simulink model "DataPath"  (R2025a)
settings: Solver=FixedStepAuto  StartTime=0  StopTime=0.02  FixedStep=1e-7  RelTol=1e-3
undefined symbols (not defined in the file): Bit_1, Bit_2, Bit_3, Bit_4, Bit_5, Bit_6, Bit_7, Bit_8
libraries: simulink_extras x126, fl_lib x34, nesl_utility x18, simulink x2
(part 6 of 7)

== system DataPath/Subsystem/ALU Regs/B2/Subsystem8 ==
  Data : Inport
  Store : Inport  Port=2
  Clock : Inport  Port=3
  Clear : Inport  Port=4
  AND : Logic  IconShape=distinctive  AllPortsSameDT=off  OutDataTypeStr=boolean
  AND1 : Logic  IconShape=distinctive  AllPortsSameDT=off  OutDataTypeStr=boolean
  D Flip-Flop : simulink_extras/Flip Flops/D Flip-Flop
  NOT : Logic  Operator=NOT  IconShape=distinctive  AllPortsSameDT=off  OutDataTypeStr=boolean
  NOT1 : Logic  Operator=NOT  IconShape=distinctive  AllPortsSameDT=off  OutDataTypeStr=boolean
  OR : Logic  Operator=OR  IconShape=distinctive  AllPortsSameDT=off  OutDataTypeStr=boolean
  Q : Outport
  !Q : Outport  Port=2
  wires:
  AND1/1 -> OR/2
  AND/1 -> OR/1
  D Flip-Flop/1 -> Q/1, AND1/2
  NOT/1 -> AND1/1
  Store/1 -> AND/2, NOT/1
  Clock/1 -> D Flip-Flop/2
  Data/1 -> AND/1
  OR/1 -> D Flip-Flop/1
  D Flip-Flop/2 -> !Q/1
  Clear/1 -> NOT1/1
  NOT1/1 -> D Flip-Flop/3

== system DataPath/Subsystem/Normalize Div/Subsystem1/Subsystem6 ==
  Data : Inport
  CLK : Inport  Port=2
  Delay One Step : Delay  DelayLength=1
  NAND{1..4} (4 alike) : Logic  Operator=NAND  IconShape=distinctive  AllPortsSameDT=off  OutDataTypeStr=boolean
  Q : Outport
  !Q : Outport  Port=2
  wires:
  NAND1/1 -> Delay One Step/1
  NAND4/1 -> NAND2/2
  Delay One Step/1 -> NAND2/1, Q/1  "Q"
  NAND2/1 -> !Q/1, NAND1/2
  NAND3/1 -> NAND4/1, NAND1/1
  CLK/1 -> NAND3/2, NAND4/2
  Data/1 -> NAND3/1

== system DataPath/Subsystem/Normalize Div/Subsystem1/Subsystem7 ==
  Data : Inport
  CLK : Inport  Port=2
  Delay One Step : Delay  DelayLength=1
  NAND{1..4} (4 alike) : Logic  Operator=NAND  IconShape=distinctive  AllPortsSameDT=off  OutDataTypeStr=boolean
  Q : Outport
  !Q : Outport  Port=2
  wires:
  NAND1/1 -> Delay One Step/1
  NAND4/1 -> NAND2/2
  Delay One Step/1 -> NAND2/1, Q/1  "Q"
  NAND2/1 -> !Q/1, NAND1/2
  NAND3/1 -> NAND4/1, NAND1/1
  CLK/1 -> NAND3/2, NAND4/2
  Data/1 -> NAND3/1

== system DataPath/Subsystem/Normalize Div/Subsystem8/Subsystem6 ==
  Data : Inport
  CLK : Inport  Port=2
  Delay One Step : Delay  DelayLength=1
  NAND{1..4} (4 alike) : Logic  Operator=NAND  IconShape=distinctive  AllPortsSameDT=off  OutDataTypeStr=boolean
  Q : Outport
  !Q : Outport  Port=2
  wires:
  NAND1/1 -> Delay One Step/1
  NAND4/1 -> NAND2/2
  Delay One Step/1 -> NAND2/1, Q/1  "Q"
  NAND2/1 -> !Q/1, NAND1/2
  NAND3/1 -> NAND4/1, NAND1/1
  CLK/1 -> NAND3/2, NAND4/2
  Data/1 -> NAND3/1

== system DataPath/Subsystem/Normalize Div/Subsystem8/Subsystem7 ==
  Data : Inport
  CLK : Inport  Port=2
  Delay One Step : Delay  DelayLength=1
  NAND{1..4} (4 alike) : Logic  Operator=NAND  IconShape=distinctive  AllPortsSameDT=off  OutDataTypeStr=boolean
  Q : Outport
  !Q : Outport  Port=2
  wires:
  NAND1/1 -> Delay One Step/1
  NAND4/1 -> NAND2/2
  Delay One Step/1 -> NAND2/1, Q/1  "Q"
  NAND2/1 -> !Q/1, NAND1/2
  NAND3/1 -> NAND4/1, NAND1/1
  CLK/1 -> NAND3/2, NAND4/2
  Data/1 -> NAND3/1

== system DataPath/Subsystem/Stepper/Subsystem1/DFF ==
  Data : Inport
  CLK : Inport  Port=2
  DLatch Master : Subsystem
  DLatch Slave : Subsystem
  NOT6 : Logic  Operator=NOT  IconShape=distinctive  AllPortsSameDT=off  OutDataTypeStr=boolean
  Q : Outport
  !Q : Outport  Port=2
  wires:
  DLatch Master/1(Q) -> DLatch Slave/1(Data)
  NOT6/1 -> DLatch Master/2(CLK)
  CLK/1 -> DLatch Slave/2(CLK), NOT6/1
  Data/1 -> DLatch Master/1(Data)
  DLatch Slave/1(Q) -> Q/1
  DLatch Slave/2(!Q) -> !Q/1

== system DataPath/Subsystem/Stepper/Subsystem2/DFF ==
  Data : Inport
  CLK : Inport  Port=2
  DLatch Master : Subsystem
  DLatch Slave : Subsystem
  NOT6 : Logic  Operator=NOT  IconShape=distinctive  AllPortsSameDT=off  OutDataTypeStr=boolean
  Q : Outport
  !Q : Outport  Port=2
  wires:
  DLatch Master/1(Q) -> DLatch Slave/1(Data)
  NOT6/1 -> DLatch Master/2(CLK)
  CLK/1 -> DLatch Slave/2(CLK), NOT6/1
  Data/1 -> DLatch Master/1(Data)
  DLatch Slave/1(Q) -> Q/1
  DLatch Slave/2(!Q) -> !Q/1

== system DataPath/Subsystem/Stepper/Subsystem3/DFF ==
  Data : Inport
  CLK : Inport  Port=2
  DLatch Master : Subsystem
  DLatch Slave : Subsystem
  NOT6 : Logic  Operator=NOT  IconShape=distinctive  AllPortsSameDT=off  OutDataTypeStr=boolean
  Q : Outport
  !Q : Outport  Port=2
  wires:
  DLatch Master/1(Q) -> DLatch Slave/1(Data)
  NOT6/1 -> DLatch Master/2(CLK)
  CLK/1 -> DLatch Slave/2(CLK), NOT6/1
  Data/1 -> DLatch Master/1(Data)
  DLatch Slave/1(Q) -> Q/1
  DLatch Slave/2(!Q) -> !Q/1

== system DataPath/Subsystem/Stepper/Subsystem4/DFF ==
  Data : Inport
  CLK : Inport  Port=2
  DLatch Master : Subsystem
  DLatch Slave : Subsystem
  NOT6 : Logic  Operator=NOT  IconShape=distinctive  AllPortsSameDT=off  OutDataTypeStr=boolean
  Q : Outport
  !Q : Outport  Port=2
  wires:
  DLatch Master/1(Q) -> DLatch Slave/1(Data)
  NOT6/1 -> DLatch Master/2(CLK)
  CLK/1 -> DLatch Slave/2(CLK), NOT6/1
  Data/1 -> DLatch Master/1(Data)
  DLatch Slave/1(Q) -> Q/1
  DLatch Slave/2(!Q) -> !Q/1

== system DataPath/Subsystem1/ALU/Adder & Logic Module/Subsystem1 ==
  Neg_A : Inport
  Carry In : Inport  Port=2
  B : Inport  Port=3
  A : Inport  Port=4
  Subtract : Inport  Port=5
  = So far : Inport  Port=6
  A>B Prev : Inport  Port=7
  !A : Logic  Operator=NOT  IconShape=distinctive  AllPortsSameDT=off  OutDataTypeStr=boolean
  !A^B : Logic  Operator=NOT  IconShape=distinctive  AllPortsSameDT=off  OutDataTypeStr=boolean
  !B : Logic  Operator=NOT  IconShape=distinctive  AllPortsSameDT=off  OutDataTypeStr=boolean
  3AND : Logic  Inputs=3  IconShape=distinctive  AllPortsSameDT=off  OutDataTypeStr=boolean
  A&&B : Logic  IconShape=distinctive  AllPortsSameDT=off  OutDataTypeStr=boolean
  A-Modifier : Logic  Operator=XOR  IconShape=distinctive  AllPortsSameDT=off  OutDataTypeStr=boolean
  ALN : Logic  Operator=OR  IconShape=distinctive  AllPortsSameDT=off  OutDataTypeStr=boolean
  A^B : Logic  Operator=XOR  IconShape=distinctive  AllPortsSameDT=off  OutDataTypeStr=boolean
  A||B : Logic  Operator=OR  IconShape=distinctive  AllPortsSameDT=off  OutDataTypeStr=boolean
  B-Modifier : Logic  Operator=XOR  IconShape=distinctive  AllPortsSameDT=off  OutDataTypeStr=boolean
  CE : Logic  IconShape=distinctive  AllPortsSameDT=off  OutDataTypeStr=boolean
  CI&&A^B : Logic  IconShape=distinctive  AllPortsSameDT=off  OutDataTypeStr=boolean
  CO|| : Logic  Operator=OR  IconShape=distinctive  AllPortsSameDT=off  OutDataTypeStr=boolean
  Mux : Mux  Inputs=6
  SUM : Logic  Operator=XOR  IconShape=distinctive  AllPortsSameDT=off  OutDataTypeStr=boolean
  Carry Out : Outport
  Bus : Outport  Port=2
  = Currently : Outport  Port=3
  A >B Next : Outport  Port=4
  wires:
  B/1 -> B-Modifier/1
  Subtract/1 -> B-Modifier/2
  CI&&A^B/1 -> CO||/1
  A&&B/1 -> Mux/2, CO||/2  "AND"
  CO||/1 -> Carry Out/1
  B-Modifier/1 -> A&&B/2, !B/1, A||B/2, A^B/2  "B_M"
  Carry In/1 -> CI&&A^B/2, SUM/2
  SUM/1 -> Mux/1  "Sum"
  A^B/1 -> Mux/4, CI&&A^B/1, 3AND/3, !A^B/1, SUM/1  "XOR"
  A>B Prev/1 -> ALN/1
  ALN/1 -> A >B Next/1
  !A^B/1 -> CE/2
  CE/1 -> = Currently/1
  3AND/1 -> ALN/2
  A-Modifier/1 -> 3AND/2, !A/1, A||B/1, A&&B/1, A^B/1
  = So far/1 -> CE/1, 3AND/1
  A||B/1 -> Mux/3  "OR"
  Mux/1 -> Bus/1
  !A/1 -> Mux/5  "!A"
  !B/1 -> Mux/6  "!B"
  A/1 -> A-Modifier/2
  Neg_A/1 -> A-Modifier/1

== system DataPath/Subsystem1/ALU/Adder & Logic Module/Subsystem2 ==
  Neg_A : Inport
  Carry In : Inport  Port=2
  B : Inport  Port=3
  A : Inport  Port=4
  Subtract : Inport  Port=5
  = So far : Inport  Port=6
  A>B Prev : Inport  Port=7
  !A : Logic  Operator=NOT  IconShape=distinctive  AllPortsSameDT=off  OutDataTypeStr=boolean
  !A^B : Logic  Operator=NOT  IconShape=distinctive  AllPortsSameDT=off  OutDataTypeStr=boolean
  !B : Logic  Operator=NOT  IconShape=distinctive  AllPortsSameDT=off  OutDataTypeStr=boolean
  3AND : Logic  Inputs=3  IconShape=distinctive  AllPortsSameDT=off  OutDataTypeStr=boolean
  A&&B : Logic  IconShape=distinctive  AllPortsSameDT=off  OutDataTypeStr=boolean
  A-Modifier : Logic  Operator=XOR  IconShape=distinctive  AllPortsSameDT=off  OutDataTypeStr=boolean
  ALN : Logic  Operator=OR  IconShape=distinctive  AllPortsSameDT=off  OutDataTypeStr=boolean
  A^B : Logic  Operator=XOR  IconShape=distinctive  AllPortsSameDT=off  OutDataTypeStr=boolean
  A||B : Logic  Operator=OR  IconShape=distinctive  AllPortsSameDT=off  OutDataTypeStr=boolean
  B-Modifier : Logic  Operator=XOR  IconShape=distinctive  AllPortsSameDT=off  OutDataTypeStr=boolean
  CE : Logic  IconShape=distinctive  AllPortsSameDT=off  OutDataTypeStr=boolean
  CI&&A^B : Logic  IconShape=distinctive  AllPortsSameDT=off  OutDataTypeStr=boolean
  CO|| : Logic  Operator=OR  IconShape=distinctive  AllPortsSameDT=off  OutDataTypeStr=boolean
  Mux : Mux  Inputs=6
  SUM : Logic  Operator=XOR  IconShape=distinctive  AllPortsSameDT=off  OutDataTypeStr=boolean
  Carry Out : Outport
  Bus : Outport  Port=2
  = Currently : Outport  Port=3
  A >B Next : Outport  Port=4
  wires:
  B/1 -> B-Modifier/1
  Subtract/1 -> B-Modifier/2
  CI&&A^B/1 -> CO||/1
  A&&B/1 -> Mux/2, CO||/2  "AND"
  CO||/1 -> Carry Out/1
  B-Modifier/1 -> A&&B/2, !B/1, A||B/2, A^B/2  "B_M"
  Carry In/1 -> CI&&A^B/2, SUM/2
  SUM/1 -> Mux/1  "Sum"
  A^B/1 -> Mux/4, CI&&A^B/1, 3AND/3, !A^B/1, SUM/1  "XOR"
  A>B Prev/1 -> ALN/1
  ALN/1 -> A >B Next/1
  !A^B/1 -> CE/2
  CE/1 -> = Currently/1
  3AND/1 -> ALN/2
  A-Modifier/1 -> 3AND/2, !A/1, A||B/1, A&&B/1, A^B/1
  = So far/1 -> CE/1, 3AND/1
  A||B/1 -> Mux/3  "OR"
  Mux/1 -> Bus/1
  !A/1 -> Mux/5  "!A"
  !B/1 -> Mux/6  "!B"
  A/1 -> A-Modifier/2
  Neg_A/1 -> A-Modifier/1

== system DataPath/Subsystem1/ALU/Adder & Logic Module/Subsystem3 ==
  Neg_A : Inport
  Carry In : Inport  Port=2
  B : Inport  Port=3
  A : Inport  Port=4
  Subtract : Inport  Port=5
  = So far : Inport  Port=6
  A>B Prev : Inport  Port=7
  !A : Logic  Operator=NOT  IconShape=distinctive  AllPortsSameDT=off  OutDataTypeStr=boolean
  !A^B : Logic  Operator=NOT  IconShape=distinctive  AllPortsSameDT=off  OutDataTypeStr=boolean
  !B : Logic  Operator=NOT  IconShape=distinctive  AllPortsSameDT=off  OutDataTypeStr=boolean
  3AND : Logic  Inputs=3  IconShape=distinctive  AllPortsSameDT=off  OutDataTypeStr=boolean
  A&&B : Logic  IconShape=distinctive  AllPortsSameDT=off  OutDataTypeStr=boolean
  A-Modifier : Logic  Operator=XOR  IconShape=distinctive  AllPortsSameDT=off  OutDataTypeStr=boolean
  ALN : Logic  Operator=OR  IconShape=distinctive  AllPortsSameDT=off  OutDataTypeStr=boolean
  A^B : Logic  Operator=XOR  IconShape=distinctive  AllPortsSameDT=off  OutDataTypeStr=boolean
  A||B : Logic  Operator=OR  IconShape=distinctive  AllPortsSameDT=off  OutDataTypeStr=boolean
  B-Modifier : Logic  Operator=XOR  IconShape=distinctive  AllPortsSameDT=off  OutDataTypeStr=boolean
  CE : Logic  IconShape=distinctive  AllPortsSameDT=off  OutDataTypeStr=boolean
  CI&&A^B : Logic  IconShape=distinctive  AllPortsSameDT=off  OutDataTypeStr=boolean
  CO|| : Logic  Operator=OR  IconShape=distinctive  AllPortsSameDT=off  OutDataTypeStr=boolean
  Mux : Mux  Inputs=6
  SUM : Logic  Operator=XOR  IconShape=distinctive  AllPortsSameDT=off  OutDataTypeStr=boolean
  Carry Out : Outport
  Bus : Outport  Port=2
  = Currently : Outport  Port=3
  A >B Next : Outport  Port=4
  wires:
  B/1 -> B-Modifier/1
  Subtract/1 -> B-Modifier/2
  CI&&A^B/1 -> CO||/1
  A&&B/1 -> Mux/2, CO||/2  "AND"
  CO||/1 -> Carry Out/1
  B-Modifier/1 -> A&&B/2, !B/1, A||B/2, A^B/2  "B_M"
  Carry In/1 -> CI&&A^B/2, SUM/2
  SUM/1 -> Mux/1  "Sum"
  A^B/1 -> Mux/4, CI&&A^B/1, 3AND/3, !A^B/1, SUM/1  "XOR"
  A>B Prev/1 -> ALN/1
  ALN/1 -> A >B Next/1
  !A^B/1 -> CE/2
  CE/1 -> = Currently/1
  3AND/1 -> ALN/2
  A-Modifier/1 -> 3AND/2, !A/1, A||B/1, A&&B/1, A^B/1
  = So far/1 -> CE/1, 3AND/1
  A||B/1 -> Mux/3  "OR"
  Mux/1 -> Bus/1
  !A/1 -> Mux/5  "!A"
  !B/1 -> Mux/6  "!B"
  A/1 -> A-Modifier/2
  Neg_A/1 -> A-Modifier/1

== system DataPath/Subsystem1/ALU/Adder & Logic Module/Subsystem4 ==
  Neg_A : Inport
  Carry In : Inport  Port=2
  B : Inport  Port=3
  A : Inport  Port=4
  Subtract : Inport  Port=5
  A>B Prev : Inport  Port=6
  = So far : Inport  Port=7
  !A : Logic  Operator=NOT  IconShape=distinctive  AllPortsSameDT=off  OutDataTypeStr=boolean
  !A^B : Logic  Operator=NOT  IconShape=distinctive  AllPortsSameDT=off  OutDataTypeStr=boolean
  !B : Logic  Operator=NOT  IconShape=distinctive  AllPortsSameDT=off  OutDataTypeStr=boolean
  3AND : Logic  Inputs=3  IconShape=distinctive  AllPortsSameDT=off  OutDataTypeStr=boolean
  A&&B : Logic  IconShape=distinctive  AllPortsSameDT=off  OutDataTypeStr=boolean
  A-Modifier : Logic  Operator=XOR  IconShape=distinctive  AllPortsSameDT=off  OutDataTypeStr=boolean
  ALN : Logic  Operator=OR  IconShape=distinctive  AllPortsSameDT=off  OutDataTypeStr=boolean
  A^B : Logic  Operator=XOR  IconShape=distinctive  AllPortsSameDT=off  OutDataTypeStr=boolean
  A||B : Logic  Operator=OR  IconShape=distinctive  AllPortsSameDT=off  OutDataTypeStr=boolean
  B-Modifier : Logic  Operator=XOR  IconShape=distinctive  AllPortsSameDT=off  OutDataTypeStr=boolean
  CE : Logic  IconShape=distinctive  AllPortsSameDT=off  OutDataTypeStr=boolean
  CI&&A^B : Logic  IconShape=distinctive  AllPortsSameDT=off  OutDataTypeStr=boolean
  CO|| : Logic  Operator=OR  IconShape=distinctive  AllPortsSameDT=off  OutDataTypeStr=boolean
  Delay One Step3 : Delay  DelayLength=1
  Mux : Mux  Inputs=6
  SUM : Logic  Operator=XOR  IconShape=distinctive  AllPortsSameDT=off  OutDataTypeStr=boolean
  Carry Out : Outport
  Bus : Outport  Port=2
  A >B Next : Outport  Port=3
  = Currently : Outport  Port=4
  wires:
  B/1 -> B-Modifier/1
  Subtract/1 -> B-Modifier/2
  CI&&A^B/1 -> CO||/1
  A&&B/1 -> Mux/2, CO||/2  "AND"
  CO||/1 -> Carry Out/1
  B-Modifier/1 -> A&&B/2, !B/1, A||B/2, A^B/2  "B_M"
  Carry In/1 -> CI&&A^B/2, SUM/2
  SUM/1 -> Mux/1  "Sum"
  A^B/1 -> Mux/4, CI&&A^B/1, 3AND/3, !A^B/1, SUM/1  "XOR"
  A>B Prev/1 -> ALN/1
  ALN/1 -> A >B Next/1
  !A^B/1 -> CE/2
  CE/1 -> = Currently/1
  3AND/1 -> ALN/2
  A-Modifier/1 -> 3AND/2, !A/1, A||B/1, A&&B/1, A^B/1
  = So far/1 -> CE/1, 3AND/1
  A||B/1 -> Mux/3  "OR"
  Mux/1 -> Delay One Step3/1
  !A/1 -> Mux/5  "!A"
  !B/1 -> Mux/6  "!B"
  A/1 -> A-Modifier/2
  Neg_A/1 -> A-Modifier/1
  Delay One Step3/1 -> Bus/1

== system DataPath/Subsystem1/ALU/Adder & Logic Module/Subsystem5 ==
  Neg_A : Inport
  Carry In : Inport  Port=2
  B : Inport  Port=3
  A : Inport  Port=4
  Subtract : Inport  Port=5
  A>B Prev : Inport  Port=6
  = So far : Inport  Port=7
  !A : Logic  Operator=NOT  IconShape=distinctive  AllPortsSameDT=off  OutDataTypeStr=boolean
  !A^B : Logic  Operator=NOT  IconShape=distinctive  AllPortsSameDT=off  OutDataTypeStr=boolean
  !B : Logic  Operator=NOT  IconShape=distinctive  AllPortsSameDT=off  OutDataTypeStr=boolean
  3AND : Logic  Inputs=3  IconShape=distinctive  AllPortsSameDT=off  OutDataTypeStr=boolean
  A&&B : Logic  IconShape=distinctive  AllPortsSameDT=off  OutDataTypeStr=boolean
  A-Modifier : Logic  Operator=XOR  IconShape=distinctive  AllPortsSameDT=off  OutDataTypeStr=boolean
  ALN : Logic  Operator=OR  IconShape=distinctive  AllPortsSameDT=off  OutDataTypeStr=boolean
  A^B : Logic  Operator=XOR  IconShape=distinctive  AllPortsSameDT=off  OutDataTypeStr=boolean
  A||B : Logic  Operator=OR  IconShape=distinctive  AllPortsSameDT=off  OutDataTypeStr=boolean
  B-Modifier : Logic  Operator=XOR  IconShape=distinctive  AllPortsSameDT=off  OutDataTypeStr=boolean
  CE : Logic  IconShape=distinctive  AllPortsSameDT=off  OutDataTypeStr=boolean
  CI&&A^B : Logic  IconShape=distinctive  AllPortsSameDT=off  OutDataTypeStr=boolean
  CO|| : Logic  Operator=OR  IconShape=distinctive  AllPortsSameDT=off  OutDataTypeStr=boolean
  Delay One Step3 : Delay  DelayLength=1
  Mux : Mux  Inputs=6
  SUM : Logic  Operator=XOR  IconShape=distinctive  AllPortsSameDT=off  OutDataTypeStr=boolean
  Carry Out : Outport
  Bus : Outport  Port=2
  A >B Next : Outport  Port=3
  = Currently : Outport  Port=4
  wires:
  B/1 -> B-Modifier/1
  Subtract/1 -> B-Modifier/2
  CI&&A^B/1 -> CO||/1
  A&&B/1 -> Mux/2, CO||/2  "AND"
  CO||/1 -> Carry Out/1
  B-Modifier/1 -> A&&B/2, !B/1, A||B/2, A^B/2  "B_M"
  Carry In/1 -> CI&&A^B/2, SUM/2
  SUM/1 -> Mux/1  "Sum"
  A^B/1 -> Mux/4, CI&&A^B/1, 3AND/3, !A^B/1, SUM/1  "XOR"
  A>B Prev/1 -> ALN/1
  ALN/1 -> A >B Next/1
  !A^B/1 -> CE/2
  CE/1 -> = Currently/1
  3AND/1 -> ALN/2
  A-Modifier/1 -> 3AND/2, !A/1, A||B/1, A&&B/1, A^B/1
  = So far/1 -> CE/1, 3AND/1
  A||B/1 -> Mux/3  "OR"
  Mux/1 -> Delay One Step3/1
  !A/1 -> Mux/5  "!A"
  !B/1 -> Mux/6  "!B"
  A/1 -> A-Modifier/2
  Neg_A/1 -> A-Modifier/1
  Delay One Step3/1 -> Bus/1

== system DataPath/Subsystem1/ALU/Adder & Logic Module/Subsystem6 ==
  Neg_A : Inport
  Carry In : Inport  Port=2
  B : Inport  Port=3
  A : Inport  Port=4
  Subtract : Inport  Port=5
  A>B Prev : Inport  Port=6
  = So far : Inport  Port=7
  !A : Logic  Operator=NOT  IconShape=distinctive  AllPortsSameDT=off  OutDataTypeStr=boolean
  !A^B : Logic  Operator=NOT  IconShape=distinctive  AllPortsSameDT=off  OutDataTypeStr=boolean
  !B : Logic  Operator=NOT  IconShape=distinctive  AllPortsSameDT=off  OutDataTypeStr=boolean
  3AND : Logic  Inputs=3  IconShape=distinctive  AllPortsSameDT=off  OutDataTypeStr=boolean
  A&&B : Logic  IconShape=distinctive  AllPortsSameDT=off  OutDataTypeStr=boolean
  A-Modifier : Logic  Operator=XOR  IconShape=distinctive  AllPortsSameDT=off  OutDataTypeStr=boolean
  ALN : Logic  Operator=OR  IconShape=distinctive  AllPortsSameDT=off  OutDataTypeStr=boolean
  A^B : Logic  Operator=XOR  IconShape=distinctive  AllPortsSameDT=off  OutDataTypeStr=boolean
  A||B : Logic  Operator=OR  IconShape=distinctive  AllPortsSameDT=off  OutDataTypeStr=boolean
  B-Modifier : Logic  Operator=XOR  IconShape=distinctive  AllPortsSameDT=off  OutDataTypeStr=boolean
  CE : Logic  IconShape=distinctive  AllPortsSameDT=off  OutDataTypeStr=boolean
  CI&&A^B : Logic  IconShape=distinctive  AllPortsSameDT=off  OutDataTypeStr=boolean
  CO|| : Logic  Operator=OR  IconShape=distinctive  AllPortsSameDT=off  OutDataTypeStr=boolean
  Delay One Step3 : Delay  DelayLength=1
  Mux : Mux  Inputs=6
  SUM : Logic  Operator=XOR  IconShape=distinctive  AllPortsSameDT=off  OutDataTypeStr=boolean
  Carry Out : Outport
  Bus : Outport  Port=2
  A >B Next : Outport  Port=3
  = Currently : Outport  Port=4
  wires:
  B/1 -> B-Modifier/1
  Subtract/1 -> B-Modifier/2
  CI&&A^B/1 -> CO||/1
  A&&B/1 -> Mux/2, CO||/2  "AND"
  CO||/1 -> Carry Out/1
  B-Modifier/1 -> A&&B/2, !B/1, A||B/2, A^B/2  "B_M"
  Carry In/1 -> CI&&A^B/2, SUM/2
  SUM/1 -> Mux/1  "Sum"
  A^B/1 -> Mux/4, CI&&A^B/1, 3AND/3, !A^B/1, SUM/1  "XOR"
  A>B Prev/1 -> ALN/1
  ALN/1 -> A >B Next/1
  !A^B/1 -> CE/2
  CE/1 -> = Currently/1
  3AND/1 -> ALN/2
  A-Modifier/1 -> 3AND/2, !A/1, A||B/1, A&&B/1, A^B/1
  = So far/1 -> CE/1, 3AND/1
  A||B/1 -> Mux/3  "OR"
  Mux/1 -> Delay One Step3/1
  !A/1 -> Mux/5  "!A"
  !B/1 -> Mux/6  "!B"
  A/1 -> A-Modifier/2
  Neg_A/1 -> A-Modifier/1
  Delay One Step3/1 -> Bus/1

== system DataPath/Subsystem1/ALU/Adder & Logic Module/Subsystem7 ==
  Neg_A : Inport
  Carry In : Inport  Port=2
  B : Inport  Port=3
  A : Inport  Port=4
  Subtract : Inport  Port=5
  A>B Prev : Inport  Port=6
  = So far : Inport  Port=7
  !A : Logic  Operator=NOT  IconShape=distinctive  AllPortsSameDT=off  OutDataTypeStr=boolean
  !A^B : Logic  Operator=NOT  IconShape=distinctive  AllPortsSameDT=off  OutDataTypeStr=boolean
  !B : Logic  Operator=NOT  IconShape=distinctive  AllPortsSameDT=off  OutDataTypeStr=boolean
  3AND : Logic  Inputs=3  IconShape=distinctive  AllPortsSameDT=off  OutDataTypeStr=boolean
  A&&B : Logic  IconShape=distinctive  AllPortsSameDT=off  OutDataTypeStr=boolean
  A-Modifier : Logic  Operator=XOR  IconShape=distinctive  AllPortsSameDT=off  OutDataTypeStr=boolean
  ALN : Logic  Operator=OR  IconShape=distinctive  AllPortsSameDT=off  OutDataTypeStr=boolean
  A^B : Logic  Operator=XOR  IconShape=distinctive  AllPortsSameDT=off  OutDataTypeStr=boolean
  A||B : Logic  Operator=OR  IconShape=distinctive  AllPortsSameDT=off  OutDataTypeStr=boolean
  B-Modifier : Logic  Operator=XOR  IconShape=distinctive  AllPortsSameDT=off  OutDataTypeStr=boolean
  CE : Logic  IconShape=distinctive  AllPortsSameDT=off  OutDataTypeStr=boolean
  CI&&A^B : Logic  IconShape=distinctive  AllPortsSameDT=off  OutDataTypeStr=boolean
  CO|| : Logic  Operator=OR  IconShape=distinctive  AllPortsSameDT=off  OutDataTypeStr=boolean
  Delay One Step3 : Delay  DelayLength=1
  Mux : Mux  Inputs=6
  SUM : Logic  Operator=XOR  IconShape=distinctive  AllPortsSameDT=off  OutDataTypeStr=boolean
  Carry Out : Outport
  Bus : Outport  Port=2
  A >B Next : Outport  Port=3
  = Currently : Outport  Port=4
  wires:
  B/1 -> B-Modifier/1
  Subtract/1 -> B-Modifier/2
  CI&&A^B/1 -> CO||/1
  A&&B/1 -> Mux/2, CO||/2  "AND"
  CO||/1 -> Carry Out/1
  B-Modifier/1 -> A&&B/2, !B/1, A||B/2, A^B/2  "B_M"
  Carry In/1 -> CI&&A^B/2, SUM/2
  SUM/1 -> Mux/1  "Sum"
  A^B/1 -> Mux/4, CI&&A^B/1, 3AND/3, !A^B/1, SUM/1  "XOR"
  A>B Prev/1 -> ALN/1
  ALN/1 -> A >B Next/1
  !A^B/1 -> CE/2
  CE/1 -> = Currently/1
  3AND/1 -> ALN/2
  A-Modifier/1 -> 3AND/2, !A/1, A||B/1, A&&B/1, A^B/1
  = So far/1 -> CE/1, 3AND/1
  A||B/1 -> Mux/3  "OR"
  Mux/1 -> Delay One Step3/1
  !A/1 -> Mux/5  "!A"
  !B/1 -> Mux/6  "!B"
  A/1 -> A-Modifier/2
  Neg_A/1 -> A-Modifier/1
  Delay One Step3/1 -> Bus/1

== system DataPath/Subsystem1/ALU/Adder & Logic Module/Subsystem8 ==
  Neg_A : Inport
  Carry In : Inport  Port=2
  B : Inport  Port=3
  A : Inport  Port=4
  Subtract : Inport  Port=5
  = So far : Inport  Port=6
  A>B Prev : Inport  Port=7
  !A : Logic  Operator=NOT  IconShape=distinctive  AllPortsSameDT=off  OutDataTypeStr=boolean
  !A^B : Logic  Operator=NOT  IconShape=distinctive  AllPortsSameDT=off  OutDataTypeStr=boolean
  !B : Logic  Operator=NOT  IconShape=distinctive  AllPortsSameDT=off  OutDataTypeStr=boolean
  3AND : Logic  Inputs=3  IconShape=distinctive  AllPortsSameDT=off  OutDataTypeStr=boolean
  A&&B : Logic  IconShape=distinctive  AllPortsSameDT=off  OutDataTypeStr=boolean
  A-Modifier : Logic  Operator=XOR  IconShape=distinctive  AllPortsSameDT=off  OutDataTypeStr=boolean
  ALN : Logic  Operator=OR  IconShape=distinctive  AllPortsSameDT=off  OutDataTypeStr=boolean
  A^B : Logic  Operator=XOR  IconShape=distinctive  AllPortsSameDT=off  OutDataTypeStr=boolean
  A||B : Logic  Operator=OR  IconShape=distinctive  AllPortsSameDT=off  OutDataTypeStr=boolean
  B-Modifier : Logic  Operator=XOR  IconShape=distinctive  AllPortsSameDT=off  OutDataTypeStr=boolean
  CE : Logic  IconShape=distinctive  AllPortsSameDT=off  OutDataTypeStr=boolean
  CI&&A^B : Logic  IconShape=distinctive  AllPortsSameDT=off  OutDataTypeStr=boolean
  CO|| : Logic  Operator=OR  IconShape=distinctive  AllPortsSameDT=off  OutDataTypeStr=boolean
  Mux : Mux  Inputs=6
  SUM : Logic  Operator=XOR  IconShape=distinctive  AllPortsSameDT=off  OutDataTypeStr=boolean
  Carry Out : Outport
  Bus : Outport  Port=2
  = Currently : Outport  Port=3
  A >B Next : Outport  Port=4
  wires:
  B/1 -> B-Modifier/1
  Subtract/1 -> B-Modifier/2
  CI&&A^B/1 -> CO||/1
  A&&B/1 -> Mux/2, CO||/2  "AND"
  CO||/1 -> Carry Out/1
  B-Modifier/1 -> A&&B/2, !B/1, A||B/2, A^B/2  "B_M"
  Carry In/1 -> CI&&A^B/2, SUM/2
  SUM/1 -> Mux/1  "Sum"
  A^B/1 -> Mux/4, CI&&A^B/1, 3AND/3, !A^B/1, SUM/1  "XOR"
  A>B Prev/1 -> ALN/1
  ALN/1 -> A >B Next/1
  !A^B/1 -> CE/2
  CE/1 -> = Currently/1
  3AND/1 -> ALN/2
  A-Modifier/1 -> 3AND/2, !A/1, A||B/1, A&&B/1, A^B/1
  = So far/1 -> CE/1, 3AND/1
  A||B/1 -> Mux/3  "OR"
  Mux/1 -> Bus/1
  !A/1 -> Mux/5  "!A"
  !B/1 -> Mux/6  "!B"
  A/1 -> A-Modifier/2
  Neg_A/1 -> A-Modifier/1

== system DataPath/Subsystem1/ALU Regs/A1/Subsystem1 ==
  Data : Inport
  Store : Inport  Port=2
  Clock : Inport  Port=3
  Clear : Inport  Port=4
  AND : Logic  IconShape=distinctive  AllPortsSameDT=off  OutDataTypeStr=boolean
  AND1 : Logic  IconShape=distinctive  AllPortsSameDT=off  OutDataTypeStr=boolean
  D Flip-Flop : simulink_extras/Flip Flops/D Flip-Flop
  NOT : Logic  Operator=NOT  IconShape=distinctive  AllPortsSameDT=off  OutDataTypeStr=boolean
  NOT1 : Logic  Operator=NOT  IconShape=distinctive  AllPortsSameDT=off  OutDataTypeStr=boolean
  OR : Logic  Operator=OR  IconShape=distinctive  AllPortsSameDT=off  OutDataTypeStr=boolean
  Q : Outport
  !Q : Outport  Port=2
  wires:
  AND1/1 -> OR/2
  AND/1 -> OR/1
  D Flip-Flop/1 -> Q/1, AND1/2
  NOT/1 -> AND1/1
  Store/1 -> AND/2, NOT/1
  Clock/1 -> D Flip-Flop/2
  Data/1 -> AND/1
  OR/1 -> D Flip-Flop/1
  D Flip-Flop/2 -> !Q/1
  Clear/1 -> NOT1/1
  NOT1/1 -> D Flip-Flop/3

== system DataPath/Subsystem1/ALU Regs/A1/Subsystem2 ==
  Data : Inport
  Store : Inport  Port=2
  Clock : Inport  Port=3
  Clear : Inport  Port=4
  AND : Logic  IconShape=distinctive  AllPortsSameDT=off  OutDataTypeStr=boolean
  AND1 : Logic  IconShape=distinctive  AllPortsSameDT=off  OutDataTypeStr=boolean
  D Flip-Flop : simulink_extras/Flip Flops/D Flip-Flop
  NOT : Logic  Operator=NOT  IconShape=distinctive  AllPortsSameDT=off  OutDataTypeStr=boolean
  NOT1 : Logic  Operator=NOT  IconShape=distinctive  AllPortsSameDT=off  OutDataTypeStr=boolean
  OR : Logic  Operator=OR  IconShape=distinctive  AllPortsSameDT=off  OutDataTypeStr=boolean
  Q : Outport
  !Q : Outport  Port=2
  wires:
  AND1/1 -> OR/2
  AND/1 -> OR/1
  D Flip-Flop/1 -> Q/1, AND1/2
  NOT/1 -> AND1/1
  Store/1 -> AND/2, NOT/1
  Clock/1 -> D Flip-Flop/2
  Data/1 -> AND/1
  OR/1 -> D Flip-Flop/1
  D Flip-Flop/2 -> !Q/1
  Clear/1 -> NOT1/1
  NOT1/1 -> D Flip-Flop/3

== system DataPath/Subsystem1/ALU Regs/A1/Subsystem3 ==
  Data : Inport
  Store : Inport  Port=2
  Clock : Inport  Port=3
  Clear : Inport  Port=4
  AND : Logic  IconShape=distinctive  AllPortsSameDT=off  OutDataTypeStr=boolean
  AND1 : Logic  IconShape=distinctive  AllPortsSameDT=off  OutDataTypeStr=boolean
  D Flip-Flop : simulink_extras/Flip Flops/D Flip-Flop
  NOT : Logic  Operator=NOT  IconShape=distinctive  AllPortsSameDT=off  OutDataTypeStr=boolean
  NOT1 : Logic  Operator=NOT  IconShape=distinctive  AllPortsSameDT=off  OutDataTypeStr=boolean
  OR : Logic  Operator=OR  IconShape=distinctive  AllPortsSameDT=off  OutDataTypeStr=boolean
  Q : Outport
  !Q : Outport  Port=2
  wires:
  AND1/1 -> OR/2
  AND/1 -> OR/1
  D Flip-Flop/1 -> Q/1, AND1/2
  NOT/1 -> AND1/1
  Store/1 -> AND/2, NOT/1
  Clock/1 -> D Flip-Flop/2
  Data/1 -> AND/1
  OR/1 -> D Flip-Flop/1
  D Flip-Flop/2 -> !Q/1
  Clear/1 -> NOT1/1
  NOT1/1 -> D Flip-Flop/3

== system DataPath/Subsystem1/ALU Regs/A1/Subsystem4 ==
  Data : Inport
  Store : Inport  Port=2
  Clock : Inport  Port=3
  Clear : Inport  Port=4
  AND : Logic  IconShape=distinctive  AllPortsSameDT=off  OutDataTypeStr=boolean
  AND1 : Logic  IconShape=distinctive  AllPortsSameDT=off  OutDataTypeStr=boolean
  D Flip-Flop : simulink_extras/Flip Flops/D Flip-Flop
  NOT : Logic  Operator=NOT  IconShape=distinctive  AllPortsSameDT=off  OutDataTypeStr=boolean
  NOT1 : Logic  Operator=NOT  IconShape=distinctive  AllPortsSameDT=off  OutDataTypeStr=boolean
  OR : Logic  Operator=OR  IconShape=distinctive  AllPortsSameDT=off  OutDataTypeStr=boolean
  Q : Outport
  !Q : Outport  Port=2
  wires:
  AND1/1 -> OR/2
  AND/1 -> OR/1
  D Flip-Flop/1 -> Q/1, AND1/2
  NOT/1 -> AND1/1
  Store/1 -> AND/2, NOT/1
  Clock/1 -> D Flip-Flop/2
  Data/1 -> AND/1
  OR/1 -> D Flip-Flop/1
  D Flip-Flop/2 -> !Q/1
  Clear/1 -> NOT1/1
  NOT1/1 -> D Flip-Flop/3

== system DataPath/Subsystem1/ALU Regs/A1/Subsystem5 ==
  Data : Inport
  Store : Inport  Port=2
  Clock : Inport  Port=3
  Clear : Inport  Port=4
  AND : Logic  IconShape=distinctive  AllPortsSameDT=off  OutDataTypeStr=boolean
  AND1 : Logic  IconShape=distinctive  AllPortsSameDT=off  OutDataTypeStr=boolean
  D Flip-Flop : simulink_extras/Flip Flops/D Flip-Flop
  NOT : Logic  Operator=NOT  IconShape=distinctive  AllPortsSameDT=off  OutDataTypeStr=boolean
  NOT1 : Logic  Operator=NOT  IconShape=distinctive  AllPortsSameDT=off  OutDataTypeStr=boolean
  OR : Logic  Operator=OR  IconShape=distinctive  AllPortsSameDT=off  OutDataTypeStr=boolean
  Q : Outport
  !Q : Outport  Port=2
  wires:
  AND1/1 -> OR/2
  AND/1 -> OR/1
  D Flip-Flop/1 -> Q/1, AND1/2
  NOT/1 -> AND1/1
  Store/1 -> AND/2, NOT/1
  Clock/1 -> D Flip-Flop/2
  Data/1 -> AND/1
  OR/1 -> D Flip-Flop/1
  D Flip-Flop/2 -> !Q/1
  Clear/1 -> NOT1/1
  NOT1/1 -> D Flip-Flop/3

== system DataPath/Subsystem1/ALU Regs/A1/Subsystem6 ==
  Data : Inport
  Store : Inport  Port=2
  Clock : Inport  Port=3
  Clear : Inport  Port=4
  AND : Logic  IconShape=distinctive  AllPortsSameDT=off  OutDataTypeStr=boolean
  AND1 : Logic  IconShape=distinctive  AllPortsSameDT=off  OutDataTypeStr=boolean
  D Flip-Flop : simulink_extras/Flip Flops/D Flip-Flop
  NOT : Logic  Operator=NOT  IconShape=distinctive  AllPortsSameDT=off  OutDataTypeStr=boolean
  NOT1 : Logic  Operator=NOT  IconShape=distinctive  AllPortsSameDT=off  OutDataTypeStr=boolean
  OR : Logic  Operator=OR  IconShape=distinctive  AllPortsSameDT=off  OutDataTypeStr=boolean
  Q : Outport
  !Q : Outport  Port=2
  wires:
  AND1/1 -> OR/2
  AND/1 -> OR/1
  D Flip-Flop/1 -> Q/1, AND1/2
  NOT/1 -> AND1/1
  Store/1 -> AND/2, NOT/1
  Clock/1 -> D Flip-Flop/2
  Data/1 -> AND/1
  OR/1 -> D Flip-Flop/1
  D Flip-Flop/2 -> !Q/1
  Clear/1 -> NOT1/1
  NOT1/1 -> D Flip-Flop/3

== system DataPath/Subsystem1/ALU Regs/A1/Subsystem7 ==
  Data : Inport
  Store : Inport  Port=2
  Clock : Inport  Port=3
  Clear : Inport  Port=4
  AND : Logic  IconShape=distinctive  AllPortsSameDT=off  OutDataTypeStr=boolean
  AND1 : Logic  IconShape=distinctive  AllPortsSameDT=off  OutDataTypeStr=boolean
  D Flip-Flop : simulink_extras/Flip Flops/D Flip-Flop
  NOT : Logic  Operator=NOT  IconShape=distinctive  AllPortsSameDT=off  OutDataTypeStr=boolean
  NOT1 : Logic  Operator=NOT  IconShape=distinctive  AllPortsSameDT=off  OutDataTypeStr=boolean
  OR : Logic  Operator=OR  IconShape=distinctive  AllPortsSameDT=off  OutDataTypeStr=boolean
  Q : Outport
  !Q : Outport  Port=2
  wires:
  AND1/1 -> OR/2
  AND/1 -> OR/1
  D Flip-Flop/1 -> Q/1, AND1/2
  NOT/1 -> AND1/1
  Store/1 -> AND/2, NOT/1
  Clock/1 -> D Flip-Flop/2
  Data/1 -> AND/1
  OR/1 -> D Flip-Flop/1
  D Flip-Flop/2 -> !Q/1
  Clear/1 -> NOT1/1
  NOT1/1 -> D Flip-Flop/3

== system DataPath/Subsystem1/ALU Regs/A1/Subsystem8 ==
  Data : Inport
  Store : Inport  Port=2
  Clock : Inport  Port=3
  Clear : Inport  Port=4
  AND : Logic  IconShape=distinctive  AllPortsSameDT=off  OutDataTypeStr=boolean
  AND1 : Logic  IconShape=distinctive  AllPortsSameDT=off  OutDataTypeStr=boolean
  D Flip-Flop : simulink_extras/Flip Flops/D Flip-Flop
  NOT : Logic  Operator=NOT  IconShape=distinctive  AllPortsSameDT=off  OutDataTypeStr=boolean
  NOT1 : Logic  Operator=NOT  IconShape=distinctive  AllPortsSameDT=off  OutDataTypeStr=boolean
  OR : Logic  Operator=OR  IconShape=distinctive  AllPortsSameDT=off  OutDataTypeStr=boolean
  Q : Outport
  !Q : Outport  Port=2
  wires:
  AND1/1 -> OR/2
  AND/1 -> OR/1
  D Flip-Flop/1 -> Q/1, AND1/2
  NOT/1 -> AND1/1
  Store/1 -> AND/2, NOT/1
  Clock/1 -> D Flip-Flop/2
  Data/1 -> AND/1
  OR/1 -> D Flip-Flop/1
  D Flip-Flop/2 -> !Q/1
  Clear/1 -> NOT1/1
  NOT1/1 -> D Flip-Flop/3

== system DataPath/Subsystem1/ALU Regs/A2/Subsystem1 ==
  Data : Inport
  Store : Inport  Port=2
  Clock : Inport  Port=3
  Clear : Inport  Port=4
  AND : Logic  IconShape=distinctive  AllPortsSameDT=off  OutDataTypeStr=boolean
  AND1 : Logic  IconShape=distinctive  AllPortsSameDT=off  OutDataTypeStr=boolean
  D Flip-Flop : simulink_extras/Flip Flops/D Flip-Flop
  NOT : Logic  Operator=NOT  IconShape=distinctive  AllPortsSameDT=off  OutDataTypeStr=boolean
  NOT1 : Logic  Operator=NOT  IconShape=distinctive  AllPortsSameDT=off  OutDataTypeStr=boolean
  OR : Logic  Operator=OR  IconShape=distinctive  AllPortsSameDT=off  OutDataTypeStr=boolean
  Q : Outport
  !Q : Outport  Port=2
  wires:
  AND1/1 -> OR/2
  AND/1 -> OR/1
  D Flip-Flop/1 -> Q/1, AND1/2
  NOT/1 -> AND1/1
  Store/1 -> AND/2, NOT/1
  Clock/1 -> D Flip-Flop/2
  Data/1 -> AND/1
  OR/1 -> D Flip-Flop/1
  D Flip-Flop/2 -> !Q/1
  Clear/1 -> NOT1/1
  NOT1/1 -> D Flip-Flop/3

== system DataPath/Subsystem1/ALU Regs/A2/Subsystem2 ==
  Data : Inport
  Store : Inport  Port=2
  Clock : Inport  Port=3
  Clear : Inport  Port=4
  AND : Logic  IconShape=distinctive  AllPortsSameDT=off  OutDataTypeStr=boolean
  AND1 : Logic  IconShape=distinctive  AllPortsSameDT=off  OutDataTypeStr=boolean
  D Flip-Flop : simulink_extras/Flip Flops/D Flip-Flop
  NOT : Logic  Operator=NOT  IconShape=distinctive  AllPortsSameDT=off  OutDataTypeStr=boolean
  NOT1 : Logic  Operator=NOT  IconShape=distinctive  AllPortsSameDT=off  OutDataTypeStr=boolean
  OR : Logic  Operator=OR  IconShape=distinctive  AllPortsSameDT=off  OutDataTypeStr=boolean
  Q : Outport
  !Q : Outport  Port=2
  wires:
  AND1/1 -> OR/2
  AND/1 -> OR/1
  D Flip-Flop/1 -> Q/1, AND1/2
  NOT/1 -> AND1/1
  Store/1 -> AND/2, NOT/1
  Clock/1 -> D Flip-Flop/2
  Data/1 -> AND/1
  OR/1 -> D Flip-Flop/1
  D Flip-Flop/2 -> !Q/1
  Clear/1 -> NOT1/1
  NOT1/1 -> D Flip-Flop/3

== system DataPath/Subsystem1/ALU Regs/A2/Subsystem3 ==
  Data : Inport
  Store : Inport  Port=2
  Clock : Inport  Port=3
  Clear : Inport  Port=4
  AND : Logic  IconShape=distinctive  AllPortsSameDT=off  OutDataTypeStr=boolean
  AND1 : Logic  IconShape=distinctive  AllPortsSameDT=off  OutDataTypeStr=boolean
  D Flip-Flop : simulink_extras/Flip Flops/D Flip-Flop
  NOT : Logic  Operator=NOT  IconShape=distinctive  AllPortsSameDT=off  OutDataTypeStr=boolean
  NOT1 : Logic  Operator=NOT  IconShape=distinctive  AllPortsSameDT=off  OutDataTypeStr=boolean
  OR : Logic  Operator=OR  IconShape=distinctive  AllPortsSameDT=off  OutDataTypeStr=boolean
  Q : Outport
  !Q : Outport  Port=2
  wires:
  AND1/1 -> OR/2
  AND/1 -> OR/1
  D Flip-Flop/1 -> Q/1, AND1/2
  NOT/1 -> AND1/1
  Store/1 -> AND/2, NOT/1
  Clock/1 -> D Flip-Flop/2
  Data/1 -> AND/1
  OR/1 -> D Flip-Flop/1
  D Flip-Flop/2 -> !Q/1
  Clear/1 -> NOT1/1
  NOT1/1 -> D Flip-Flop/3

== system DataPath/Subsystem1/ALU Regs/A2/Subsystem4 ==
  Data : Inport
  Store : Inport  Port=2
  Clock : Inport  Port=3
  Clear : Inport  Port=4
  AND : Logic  IconShape=distinctive  AllPortsSameDT=off  OutDataTypeStr=boolean
  AND1 : Logic  IconShape=distinctive  AllPortsSameDT=off  OutDataTypeStr=boolean
  D Flip-Flop : simulink_extras/Flip Flops/D Flip-Flop
  NOT : Logic  Operator=NOT  IconShape=distinctive  AllPortsSameDT=off  OutDataTypeStr=boolean
  NOT1 : Logic  Operator=NOT  IconShape=distinctive  AllPortsSameDT=off  OutDataTypeStr=boolean
  OR : Logic  Operator=OR  IconShape=distinctive  AllPortsSameDT=off  OutDataTypeStr=boolean
  Q : Outport
  !Q : Outport  Port=2
  wires:
  AND1/1 -> OR/2
  AND/1 -> OR/1
  D Flip-Flop/1 -> Q/1, AND1/2
  NOT/1 -> AND1/1
  Store/1 -> AND/2, NOT/1
  Clock/1 -> D Flip-Flop/2
  Data/1 -> AND/1
  OR/1 -> D Flip-Flop/1
  D Flip-Flop/2 -> !Q/1
  Clear/1 -> NOT1/1
  NOT1/1 -> D Flip-Flop/3

== system DataPath/Subsystem1/ALU Regs/A2/Subsystem5 ==
  Data : Inport
  Store : Inport  Port=2
  Clock : Inport  Port=3
  Clear : Inport  Port=4
  AND : Logic  IconShape=distinctive  AllPortsSameDT=off  OutDataTypeStr=boolean
  AND1 : Logic  IconShape=distinctive  AllPortsSameDT=off  OutDataTypeStr=boolean
  D Flip-Flop : simulink_extras/Flip Flops/D Flip-Flop
  NOT : Logic  Operator=NOT  IconShape=distinctive  AllPortsSameDT=off  OutDataTypeStr=boolean
  NOT1 : Logic  Operator=NOT  IconShape=distinctive  AllPortsSameDT=off  OutDataTypeStr=boolean
  OR : Logic  Operator=OR  IconShape=distinctive  AllPortsSameDT=off  OutDataTypeStr=boolean
  Q : Outport
  !Q : Outport  Port=2
  wires:
  AND1/1 -> OR/2
  AND/1 -> OR/1
  D Flip-Flop/1 -> Q/1, AND1/2
  NOT/1 -> AND1/1
  Store/1 -> AND/2, NOT/1
  Clock/1 -> D Flip-Flop/2
  Data/1 -> AND/1
  OR/1 -> D Flip-Flop/1
  D Flip-Flop/2 -> !Q/1
  Clear/1 -> NOT1/1
  NOT1/1 -> D Flip-Flop/3

== system DataPath/Subsystem1/ALU Regs/A2/Subsystem6 ==
  Data : Inport
  Store : Inport  Port=2
  Clock : Inport  Port=3
  Clear : Inport  Port=4
  AND : Logic  IconShape=distinctive  AllPortsSameDT=off  OutDataTypeStr=boolean
  AND1 : Logic  IconShape=distinctive  AllPortsSameDT=off  OutDataTypeStr=boolean
  D Flip-Flop : simulink_extras/Flip Flops/D Flip-Flop
  NOT : Logic  Operator=NOT  IconShape=distinctive  AllPortsSameDT=off  OutDataTypeStr=boolean
  NOT1 : Logic  Operator=NOT  IconShape=distinctive  AllPortsSameDT=off  OutDataTypeStr=boolean
  OR : Logic  Operator=OR  IconShape=distinctive  AllPortsSameDT=off  OutDataTypeStr=boolean
  Q : Outport
  !Q : Outport  Port=2
  wires:
  AND1/1 -> OR/2
  AND/1 -> OR/1
  D Flip-Flop/1 -> Q/1, AND1/2
  NOT/1 -> AND1/1
  Store/1 -> AND/2, NOT/1
  Clock/1 -> D Flip-Flop/2
  Data/1 -> AND/1
  OR/1 -> D Flip-Flop/1
  D Flip-Flop/2 -> !Q/1
  Clear/1 -> NOT1/1
  NOT1/1 -> D Flip-Flop/3

== system DataPath/Subsystem1/ALU Regs/A2/Subsystem7 ==
  Data : Inport
  Store : Inport  Port=2
  Clock : Inport  Port=3
  Clear : Inport  Port=4
  AND : Logic  IconShape=distinctive  AllPortsSameDT=off  OutDataTypeStr=boolean
  AND1 : Logic  IconShape=distinctive  AllPortsSameDT=off  OutDataTypeStr=boolean
  D Flip-Flop : simulink_extras/Flip Flops/D Flip-Flop
  NOT : Logic  Operator=NOT  IconShape=distinctive  AllPortsSameDT=off  OutDataTypeStr=boolean
  NOT1 : Logic  Operator=NOT  IconShape=distinctive  AllPortsSameDT=off  OutDataTypeStr=boolean
  OR : Logic  Operator=OR  IconShape=distinctive  AllPortsSameDT=off  OutDataTypeStr=boolean
  Q : Outport
  !Q : Outport  Port=2
  wires:
  AND1/1 -> OR/2
  AND/1 -> OR/1
  D Flip-Flop/1 -> Q/1, AND1/2
  NOT/1 -> AND1/1
  Store/1 -> AND/2, NOT/1
  Clock/1 -> D Flip-Flop/2
  Data/1 -> AND/1
  OR/1 -> D Flip-Flop/1
  D Flip-Flop/2 -> !Q/1
  Clear/1 -> NOT1/1
  NOT1/1 -> D Flip-Flop/3

== system DataPath/Subsystem1/ALU Regs/A2/Subsystem8 ==
  Data : Inport
  Store : Inport  Port=2
  Clock : Inport  Port=3
  Clear : Inport  Port=4
  AND : Logic  IconShape=distinctive  AllPortsSameDT=off  OutDataTypeStr=boolean
  AND1 : Logic  IconShape=distinctive  AllPortsSameDT=off  OutDataTypeStr=boolean
  D Flip-Flop : simulink_extras/Flip Flops/D Flip-Flop
  NOT : Logic  Operator=NOT  IconShape=distinctive  AllPortsSameDT=off  OutDataTypeStr=boolean
  NOT1 : Logic  Operator=NOT  IconShape=distinctive  AllPortsSameDT=off  OutDataTypeStr=boolean
  OR : Logic  Operator=OR  IconShape=distinctive  AllPortsSameDT=off  OutDataTypeStr=boolean
  Q : Outport
  !Q : Outport  Port=2
  wires:
  AND1/1 -> OR/2
  AND/1 -> OR/1
  D Flip-Flop/1 -> Q/1, AND1/2
  NOT/1 -> AND1/1
  Store/1 -> AND/2, NOT/1
  Clock/1 -> D Flip-Flop/2
  Data/1 -> AND/1
  OR/1 -> D Flip-Flop/1
  D Flip-Flop/2 -> !Q/1
  Clear/1 -> NOT1/1
  NOT1/1 -> D Flip-Flop/3

== system DataPath/Subsystem1/ALU Regs/B1/Subsystem1 ==
  Data : Inport
  Store : Inport  Port=2
  Clock : Inport  Port=3
  Clear : Inport  Port=4
  AND : Logic  IconShape=distinctive  AllPortsSameDT=off  OutDataTypeStr=boolean
  AND1 : Logic  IconShape=distinctive  AllPortsSameDT=off  OutDataTypeStr=boolean
  D Flip-Flop : simulink_extras/Flip Flops/D Flip-Flop
  NOT : Logic  Operator=NOT  IconShape=distinctive  AllPortsSameDT=off  OutDataTypeStr=boolean
  NOT1 : Logic  Operator=NOT  IconShape=distinctive  AllPortsSameDT=off  OutDataTypeStr=boolean
  OR : Logic  Operator=OR  IconShape=distinctive  AllPortsSameDT=off  OutDataTypeStr=boolean
  Q : Outport
  !Q : Outport  Port=2
  wires:
  AND1/1 -> OR/2
  AND/1 -> OR/1
  D Flip-Flop/1 -> Q/1, AND1/2
  NOT/1 -> AND1/1
  Store/1 -> AND/2, NOT/1
  Clock/1 -> D Flip-Flop/2
  Data/1 -> AND/1
  OR/1 -> D Flip-Flop/1
  D Flip-Flop/2 -> !Q/1
  Clear/1 -> NOT1/1
  NOT1/1 -> D Flip-Flop/3

== system DataPath/Subsystem1/ALU Regs/B1/Subsystem2 ==
  Data : Inport
  Store : Inport  Port=2
  Clock : Inport  Port=3
  Clear : Inport  Port=4
  AND : Logic  IconShape=distinctive  AllPortsSameDT=off  OutDataTypeStr=boolean
  AND1 : Logic  IconShape=distinctive  AllPortsSameDT=off  OutDataTypeStr=boolean
  D Flip-Flop : simulink_extras/Flip Flops/D Flip-Flop
  NOT : Logic  Operator=NOT  IconShape=distinctive  AllPortsSameDT=off  OutDataTypeStr=boolean
  NOT1 : Logic  Operator=NOT  IconShape=distinctive  AllPortsSameDT=off  OutDataTypeStr=boolean
  OR : Logic  Operator=OR  IconShape=distinctive  AllPortsSameDT=off  OutDataTypeStr=boolean
  Q : Outport
  !Q : Outport  Port=2
  wires:
  AND1/1 -> OR/2
  AND/1 -> OR/1
  D Flip-Flop/1 -> Q/1, AND1/2
  NOT/1 -> AND1/1
  Store/1 -> AND/2, NOT/1
  Clock/1 -> D Flip-Flop/2
  Data/1 -> AND/1
  OR/1 -> D Flip-Flop/1
  D Flip-Flop/2 -> !Q/1
  Clear/1 -> NOT1/1
  NOT1/1 -> D Flip-Flop/3

== system DataPath/Subsystem1/ALU Regs/B1/Subsystem3 ==
  Data : Inport
  Store : Inport  Port=2
  Clock : Inport  Port=3
  Clear : Inport  Port=4
  AND : Logic  IconShape=distinctive  AllPortsSameDT=off  OutDataTypeStr=boolean
  AND1 : Logic  IconShape=distinctive  AllPortsSameDT=off  OutDataTypeStr=boolean
  D Flip-Flop : simulink_extras/Flip Flops/D Flip-Flop
  NOT : Logic  Operator=NOT  IconShape=distinctive  AllPortsSameDT=off  OutDataTypeStr=boolean
  NOT1 : Logic  Operator=NOT  IconShape=distinctive  AllPortsSameDT=off  OutDataTypeStr=boolean
  OR : Logic  Operator=OR  IconShape=distinctive  AllPortsSameDT=off  OutDataTypeStr=boolean
  Q : Outport
  !Q : Outport  Port=2
  wires:
  AND1/1 -> OR/2
  AND/1 -> OR/1
  D Flip-Flop/1 -> Q/1, AND1/2
  NOT/1 -> AND1/1
  Store/1 -> AND/2, NOT/1
  Clock/1 -> D Flip-Flop/2
  Data/1 -> AND/1
  OR/1 -> D Flip-Flop/1
  D Flip-Flop/2 -> !Q/1
  Clear/1 -> NOT1/1
  NOT1/1 -> D Flip-Flop/3

== system DataPath/Subsystem1/ALU Regs/B1/Subsystem4 ==
  Data : Inport
  Store : Inport  Port=2
  Clock : Inport  Port=3
  Clear : Inport  Port=4
  AND : Logic  IconShape=distinctive  AllPortsSameDT=off  OutDataTypeStr=boolean
  AND1 : Logic  IconShape=distinctive  AllPortsSameDT=off  OutDataTypeStr=boolean
  D Flip-Flop : simulink_extras/Flip Flops/D Flip-Flop
  NOT : Logic  Operator=NOT  IconShape=distinctive  AllPortsSameDT=off  OutDataTypeStr=boolean
  NOT1 : Logic  Operator=NOT  IconShape=distinctive  AllPortsSameDT=off  OutDataTypeStr=boolean
  OR : Logic  Operator=OR  IconShape=distinctive  AllPortsSameDT=off  OutDataTypeStr=boolean
  Q : Outport
  !Q : Outport  Port=2
  wires:
  AND1/1 -> OR/2
  AND/1 -> OR/1
  D Flip-Flop/1 -> Q/1, AND1/2
  NOT/1 -> AND1/1
  Store/1 -> AND/2, NOT/1
  Clock/1 -> D Flip-Flop/2
  Data/1 -> AND/1
  OR/1 -> D Flip-Flop/1
  D Flip-Flop/2 -> !Q/1
  Clear/1 -> NOT1/1
  NOT1/1 -> D Flip-Flop/3

== system DataPath/Subsystem1/ALU Regs/B1/Subsystem5 ==
  Data : Inport
  Store : Inport  Port=2
  Clock : Inport  Port=3
  Clear : Inport  Port=4
  AND : Logic  IconShape=distinctive  AllPortsSameDT=off  OutDataTypeStr=boolean
  AND1 : Logic  IconShape=distinctive  AllPortsSameDT=off  OutDataTypeStr=boolean
  D Flip-Flop : simulink_extras/Flip Flops/D Flip-Flop
  NOT : Logic  Operator=NOT  IconShape=distinctive  AllPortsSameDT=off  OutDataTypeStr=boolean
  NOT1 : Logic  Operator=NOT  IconShape=distinctive  AllPortsSameDT=off  OutDataTypeStr=boolean
  OR : Logic  Operator=OR  IconShape=distinctive  AllPortsSameDT=off  OutDataTypeStr=boolean
  Q : Outport
  !Q : Outport  Port=2
  wires:
  AND1/1 -> OR/2
  AND/1 -> OR/1
  D Flip-Flop/1 -> Q/1, AND1/2
  NOT/1 -> AND1/1
  Store/1 -> AND/2, NOT/1
  Clock/1 -> D Flip-Flop/2
  Data/1 -> AND/1
  OR/1 -> D Flip-Flop/1
  D Flip-Flop/2 -> !Q/1
  Clear/1 -> NOT1/1
  NOT1/1 -> D Flip-Flop/3

== system DataPath/Subsystem1/ALU Regs/B1/Subsystem6 ==
  Data : Inport
  Store : Inport  Port=2
  Clock : Inport  Port=3
  Clear : Inport  Port=4
  AND : Logic  IconShape=distinctive  AllPortsSameDT=off  OutDataTypeStr=boolean
  AND1 : Logic  IconShape=distinctive  AllPortsSameDT=off  OutDataTypeStr=boolean
  D Flip-Flop : simulink_extras/Flip Flops/D Flip-Flop
  NOT : Logic  Operator=NOT  IconShape=distinctive  AllPortsSameDT=off  OutDataTypeStr=boolean
  NOT1 : Logic  Operator=NOT  IconShape=distinctive  AllPortsSameDT=off  OutDataTypeStr=boolean
  OR : Logic  Operator=OR  IconShape=distinctive  AllPortsSameDT=off  OutDataTypeStr=boolean
  Q : Outport
  !Q : Outport  Port=2
  wires:
  AND1/1 -> OR/2
  AND/1 -> OR/1
  D Flip-Flop/1 -> Q/1, AND1/2
  NOT/1 -> AND1/1
  Store/1 -> AND/2, NOT/1
  Clock/1 -> D Flip-Flop/2
  Data/1 -> AND/1
  OR/1 -> D Flip-Flop/1
  D Flip-Flop/2 -> !Q/1
  Clear/1 -> NOT1/1
  NOT1/1 -> D Flip-Flop/3

== system DataPath/Subsystem1/ALU Regs/B1/Subsystem7 ==
  Data : Inport
  Store : Inport  Port=2
  Clock : Inport  Port=3
  Clear : Inport  Port=4
  AND : Logic  IconShape=distinctive  AllPortsSameDT=off  OutDataTypeStr=boolean
  AND1 : Logic  IconShape=distinctive  AllPortsSameDT=off  OutDataTypeStr=boolean
  D Flip-Flop : simulink_extras/Flip Flops/D Flip-Flop
  NOT : Logic  Operator=NOT  IconShape=distinctive  AllPortsSameDT=off  OutDataTypeStr=boolean
  NOT1 : Logic  Operator=NOT  IconShape=distinctive  AllPortsSameDT=off  OutDataTypeStr=boolean
  OR : Logic  Operator=OR  IconShape=distinctive  AllPortsSameDT=off  OutDataTypeStr=boolean
  Q : Outport
  !Q : Outport  Port=2
  wires:
  AND1/1 -> OR/2
  AND/1 -> OR/1
  D Flip-Flop/1 -> Q/1, AND1/2
  NOT/1 -> AND1/1
  Store/1 -> AND/2, NOT/1
  Clock/1 -> D Flip-Flop/2
  Data/1 -> AND/1
  OR/1 -> D Flip-Flop/1
  D Flip-Flop/2 -> !Q/1
  Clear/1 -> NOT1/1
  NOT1/1 -> D Flip-Flop/3

== system DataPath/Subsystem1/ALU Regs/B1/Subsystem8 ==
  Data : Inport
  Store : Inport  Port=2
  Clock : Inport  Port=3
  Clear : Inport  Port=4
  AND : Logic  IconShape=distinctive  AllPortsSameDT=off  OutDataTypeStr=boolean
  AND1 : Logic  IconShape=distinctive  AllPortsSameDT=off  OutDataTypeStr=boolean
  D Flip-Flop : simulink_extras/Flip Flops/D Flip-Flop
  NOT : Logic  Operator=NOT  IconShape=distinctive  AllPortsSameDT=off  OutDataTypeStr=boolean
  NOT1 : Logic  Operator=NOT  IconShape=distinctive  AllPortsSameDT=off  OutDataTypeStr=boolean
  OR : Logic  Operator=OR  IconShape=distinctive  AllPortsSameDT=off  OutDataTypeStr=boolean
  Q : Outport
  !Q : Outport  Port=2
  wires:
  AND1/1 -> OR/2
  AND/1 -> OR/1
  D Flip-Flop/1 -> Q/1, AND1/2
  NOT/1 -> AND1/1
  Store/1 -> AND/2, NOT/1
  Clock/1 -> D Flip-Flop/2
  Data/1 -> AND/1
  OR/1 -> D Flip-Flop/1
  D Flip-Flop/2 -> !Q/1
  Clear/1 -> NOT1/1
  NOT1/1 -> D Flip-Flop/3

== system DataPath/Subsystem1/ALU Regs/B2/Subsystem1 ==
  Data : Inport
  Store : Inport  Port=2
  Clock : Inport  Port=3
  Clear : Inport  Port=4
  AND : Logic  IconShape=distinctive  AllPortsSameDT=off  OutDataTypeStr=boolean
  AND1 : Logic  IconShape=distinctive  AllPortsSameDT=off  OutDataTypeStr=boolean
  D Flip-Flop : simulink_extras/Flip Flops/D Flip-Flop
  NOT : Logic  Operator=NOT  IconShape=distinctive  AllPortsSameDT=off  OutDataTypeStr=boolean
  NOT1 : Logic  Operator=NOT  IconShape=distinctive  AllPortsSameDT=off  OutDataTypeStr=boolean
  OR : Logic  Operator=OR  IconShape=distinctive  AllPortsSameDT=off  OutDataTypeStr=boolean
  Q : Outport
  !Q : Outport  Port=2
  wires:
  AND1/1 -> OR/2
  AND/1 -> OR/1
  D Flip-Flop/1 -> Q/1, AND1/2
  NOT/1 -> AND1/1
  Store/1 -> AND/2, NOT/1
  Clock/1 -> D Flip-Flop/2
  Data/1 -> AND/1
  OR/1 -> D Flip-Flop/1
  D Flip-Flop/2 -> !Q/1
  Clear/1 -> NOT1/1
  NOT1/1 -> D Flip-Flop/3

== system DataPath/Subsystem1/ALU Regs/B2/Subsystem2 ==
  Data : Inport
  Store : Inport  Port=2
  Clock : Inport  Port=3
  Clear : Inport  Port=4
  AND : Logic  IconShape=distinctive  AllPortsSameDT=off  OutDataTypeStr=boolean
  AND1 : Logic  IconShape=distinctive  AllPortsSameDT=off  OutDataTypeStr=boolean
  D Flip-Flop : simulink_extras/Flip Flops/D Flip-Flop
  NOT : Logic  Operator=NOT  IconShape=distinctive  AllPortsSameDT=off  OutDataTypeStr=boolean
  NOT1 : Logic  Operator=NOT  IconShape=distinctive  AllPortsSameDT=off  OutDataTypeStr=boolean
  OR : Logic  Operator=OR  IconShape=distinctive  AllPortsSameDT=off  OutDataTypeStr=boolean
  Q : Outport
  !Q : Outport  Port=2
  wires:
  AND1/1 -> OR/2
  AND/1 -> OR/1
  D Flip-Flop/1 -> Q/1, AND1/2
  NOT/1 -> AND1/1
  Store/1 -> AND/2, NOT/1
  Clock/1 -> D Flip-Flop/2
  Data/1 -> AND/1
  OR/1 -> D Flip-Flop/1
  D Flip-Flop/2 -> !Q/1
  Clear/1 -> NOT1/1
  NOT1/1 -> D Flip-Flop/3

== system DataPath/Subsystem1/ALU Regs/B2/Subsystem3 ==
  Data : Inport
  Store : Inport  Port=2
  Clock : Inport  Port=3
  Clear : Inport  Port=4
  AND : Logic  IconShape=distinctive  AllPortsSameDT=off  OutDataTypeStr=boolean
  AND1 : Logic  IconShape=distinctive  AllPortsSameDT=off  OutDataTypeStr=boolean
  D Flip-Flop : simulink_extras/Flip Flops/D Flip-Flop
  NOT : Logic  Operator=NOT  IconShape=distinctive  AllPortsSameDT=off  OutDataTypeStr=boolean
  NOT1 : Logic  Operator=NOT  IconShape=distinctive  AllPortsSameDT=off  OutDataTypeStr=boolean
  OR : Logic  Operator=OR  IconShape=distinctive  AllPortsSameDT=off  OutDataTypeStr=boolean
  Q : Outport
  !Q : Outport  Port=2
  wires:
  AND1/1 -> OR/2
  AND/1 -> OR/1
  D Flip-Flop/1 -> Q/1, AND1/2
  NOT/1 -> AND1/1
  Store/1 -> AND/2, NOT/1
  Clock/1 -> D Flip-Flop/2
  Data/1 -> AND/1
  OR/1 -> D Flip-Flop/1
  D Flip-Flop/2 -> !Q/1
  Clear/1 -> NOT1/1
  NOT1/1 -> D Flip-Flop/3
